simulink model "simlab8a"  (R2021a)
settings: Solver=ode4  StartTime=0.0  StopTime=max(T)  FixedStep=0.001  RelTol=1e-3
values from neighbouring files (symbols this model uses):
  B1 = Bm+N^2*BL    (= 0.000665881525719)    [cslab8.m]
  J = Jm+N^2*JL    (= 0.000197449330572)    [cslab8.m]
  K = KT/Ra    (= 0.0210465116279)    [cslab8.m]
  K1 = wn^2*J/(Kp*K)    [cslab8.m]
  K2 = (2*zt*wn*J-B)/(K*KTG)    [cslab8.m]
  KB = 0.181    [cslab8.m]
  Kp = 0.36    [cslab8.m]
  KTG = 0.1    [cslab8.m]
  thm_lmt = 4*398*pi/180    (= 27.7856416917)    [cslab8.m]
libraries: simulink x1
settings Model: Creator=martinsundar  LastModifiedBy=martinsundar

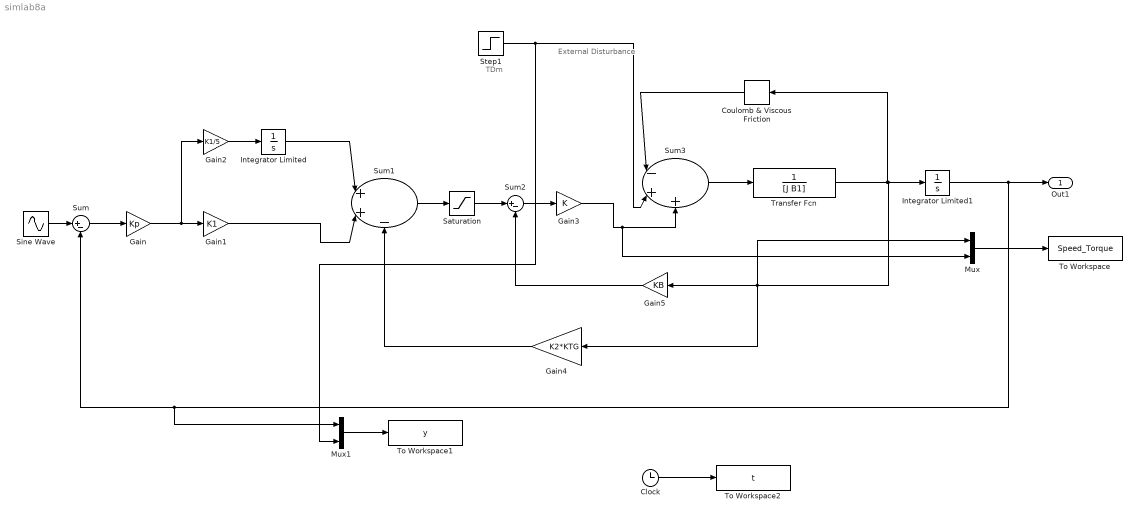
== system simlab8a ==
  note: External Disturbance
  note: TDm
  Clock : Clock
  Coulomb & Viscous Friction : simulink/Discontinuities/Coulomb & Viscous Friction  offset=0.06  gain=0
  Gain : Gain  Gain=Kp
  Gain1 : Gain  Gain=K1
  Gain2 : Gain  Gain=K1/5
  Gain3 : Gain  Gain=K
  Gain4 : Gain  Gain=K2*KTG
  Gain5 : Gain  Gain=KB
  Integrator Limited : Integrator  LimitOutput=on  UpperSaturationLimit=13  LowerSaturationLimit=-13
  Integrator Limited1 : Integrator  LimitOutput=on  UpperSaturationLimit=thm_lmt  LowerSaturationLimit=-thm_lmt
  Mux : Mux  Inputs=2
  Mux1 : Mux  Inputs=2
  Saturation : Saturate  UpperLimit=28  LowerLimit=-28
  Sine Wave : Sin  Amplitude=0.1*4*pi*398/180  Frequency=10*pi  SampleTime=0
  Step1 : Step  Time=0  After=0  SampleTime=0
  Sum : Sum  Inputs=|+-
  Sum1 : Sum  Inputs=|++-
  Sum2 : Sum  Inputs=|+-
  Sum3 : Sum  Inputs=|-++
  To Workspace : ToWorkspace  VariableName=Speed_Torque  SampleTime=-1
  To Workspace1 : ToWorkspace  VariableName=y  SampleTime=-1
  To Workspace2 : ToWorkspace  VariableName=t  SampleTime=-1
  Transfer Fcn : TransferFcn  Denominator=[J B1]
  Out1 : Outport
  wires:
  Sum/1 -> Gain/1
  Gain/1 -> Gain2/1, Gain1/1
  Gain2/1 -> Integrator Limited/1
  Gain1/1 -> Sum1/2
  Integrator Limited/1 -> Sum1/1
  Sum1/1 -> Saturation/1
  Saturation/1 -> Sum2/1
  Sum2/1 -> Gain3/1
  Gain4/1 -> Sum1/3
  Gain5/1 -> Sum2/2
  Gain3/1 -> Mux/2, Sum3/3
  Step1/1 -> Mux1/2, Sum3/2
  Sum3/1 -> Transfer Fcn/1
  Transfer Fcn/1 -> Coulomb & Viscous Friction/1, Gain4/1, Mux/1, Gain5/1, Integrator Limited1/1
  Coulomb & Viscous Friction/1 -> Sum3/1
  Integrator Limited1/1 -> Out1/1, Mux1/1, Sum/2
  Mux/1 -> To Workspace/1
  Mux1/1 -> To Workspace1/1
  Clock/1 -> To Workspace2/1
  Sine Wave/1 -> Sum/1
